simulink model "5_R_triggering"  (R2014a)
settings: Solver=ode23t  StartTime=0.0  StopTime=0.04  RelTol=1e-6
libraries: powerlib x11
settings Model: Creator=CHANDRA BABU  LastModifiedBy=Divya M
settings SolverCC: ZeroCrossControl=DisableAll
settings DataIOCC: SignalLoggingSaveFormat=ModelDataLogs
settings OptimizationCC: ExpressionDepthLimit=2147483647
settings DebuggingCC: UnderspecifiedInitializationDetection=Classic  FcnCallInpInsideContextMsg=UseLocalSettings  StateNameClashWarn=warning
settings GRTTargetCC: CombineOutputUpdateFcns=off  GRTInterface=on

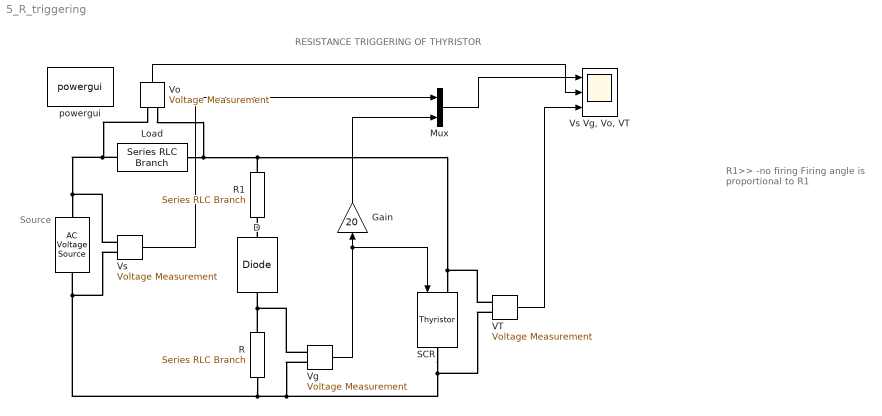
== system 5_R_triggering ==
  note: RESISTANCE TRIGGERING OF THYRISTOR
  note: R1>> -no firing
      | Firing angle is proportional to R1
  note: Source
  " " : powerlib/Electrical Sources/AC Voltage Source  Amplitude=100  Phase=0  Frequency=50  SampleTime=0  Measurements=None
  D : powerlib/Power Electronics/Diode  Ron=0.001  Lon=0  Vf=0  IC=0  UseSnubber=off  Rs=500  Cs=250e-9  Measurements=off
  Gain : Gain  Gain=20
  Load : powerlib/Elements/Series RLC Branch  LConnTagsString=__new0  RConnTagsString=__new0  BranchType=R  Resistance=2.5  Inductance=1e-3  SetiL0=off  InitialCurrent=0  Capacitance=1e-6  Setx0=off  InitialVoltage=0  Measurements=None
  Mux : Mux  Inputs=2
  R : powerlib/Elements/Series RLC Branch  LConnTagsString=__new0  RConnTagsString=__new0  BranchType=R  Resistance=5  Inductance=1e-3  SetiL0=off  InitialCurrent=0  Capacitance=1e-6  Setx0=off  InitialVoltage=0  Measurements=None
  R1 : powerlib/Elements/Series RLC Branch  LConnTagsString=__new0  RConnTagsString=__new0  BranchType=R  Resistance=350  Inductance=1e-3  SetiL0=off  InitialCurrent=0  Capacitance=1e-6  Setx0=off  InitialVoltage=0  Measurements=None
  SCR : powerlib/Power Electronics/Thyristor  Ron=0.001  Lon=0  Vf=0.8  IC=0  Rs=500  Cs=250e-9  Measurements=off
  VT : powerlib/Measurements/Voltage Measurement  PhasorSimulation=off  OutputType=Complex  PSBequivalent=0
  Vg : powerlib/Measurements/Voltage Measurement  PhasorSimulation=off  OutputType=Complex  PSBequivalent=0
  Vo : powerlib/Measurements/Voltage Measurement  PhasorSimulation=off  OutputType=Complex  PSBequivalent=0
  Vs : powerlib/Measurements/Voltage Measurement  PhasorSimulation=off  OutputType=Complex  PSBequivalent=0
  "Vs Vg, Vo, VT" : Scope  NumInputPorts=3
      settings: YMin=-100~-100~-100  YMax=100~100~100  SaveName=Outputvoltage1
  powergui : powerlib/powergui  Priority=1  SimulationMode=Continuous  SolverType=Tustin  SampleTime=50e-6  frequency=60  SPID=off  DisableSnubberDevices=off  DisableRonSwitches=off  DisableVfSwitches=off  SwTol=0  Interpol=off  DisplayEquations=off  Ts=0  methode=off  frequencyindice=0  Pbase=100e6  ErrMax=1e-4  Iterations=50  UnitsV=kV  UnitsW=MW  FunctionMessages=off  echomessages=off  HookPort=off  EnableUseOfTLC=off  x0status=blocks  RestoreLinks=warning  ResistiveCurrentMeasurement=off  Frange=[0:2:500]  Ylog=off  Xlog=on  ShowGrid=off  save=off  variable=ZData  structure=Outputvoltage  ZoomFFT=on  StartTime=0.0  cycles=1  DisplayStyle=1  fundamental=50  FreqAxis=on  MaxFrequency=1000  frequencyindicesteady=1  RmsSteady=1  display=off
  wires:
  Mux/1 -> "Vs Vg, Vo, VT"/1
  Vg/1 -> SCR/1, Gain/1
  Gain/1 -> Mux/2
  Vs/1 -> Mux/1
  VT/1 -> "Vs Vg, Vo, VT"/3
  Vo/1 -> "Vs Vg, Vo, VT"/2
  connections:
  Load/RConn1 -- Vs/LConn1 -- " "/RConn1 -- Vo/LConn1
  Load/LConn1 -- Vo/LConn2 -- R1/RConn1 -- VT/LConn1 -- SCR/LConn1
  SCR/RConn1 -- Vs/LConn2 -- " "/LConn1 -- R/LConn1 -- Vg/LConn2 -- VT/LConn2
  R/RConn1 -- D/RConn1 -- Vg/LConn1
  D/LConn1 -- R1/LConn1
